simulink model "Kidney_Insulin36"  (R2018a)
settings: Solver=VariableStepAuto  StartTime=0.0  StopTime=10.0  RelTol=1e-3
undefined symbols (not defined in the file): Q_i_K, V_i_K
settings Model: Creator=cgonterman  LastModifiedBy=cgonterman

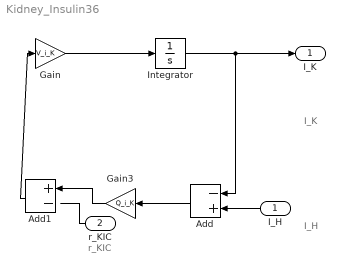
== system Kidney_Insulin36 ==
  note: I_H
  note: r_KIC
  note: I_K
  "I_H " : Inport
  "r_KIC " : Inport  Port=2
  Add : Sum  Inputs=-+
  Add1 : Sum  Inputs=+-
  Gain : Gain  Gain=V_i_K
  Gain3 : Gain  Gain=Q_i_K
  Integrator : Integrator
  "I_K " : Outport
  wires:
  "r_KIC "/1 -> ?
  Integrator/1 -> Add/1, "I_K "/1
  Gain/1 -> Integrator/1
  "I_H "/1 -> Add/2
  Add/1 -> Gain3/1
  Gain3/1 -> Add1/1
  Add1/1 -> Gain/1
